simulink model "vanilla_RNN_layer"  (R2025b)
settings: Solver=ode4  StartTime=0.0  StopTime=10.0  FixedStep=1e-3  RelTol=1e-3
settings Model: Creator=llp  LastModifiedBy=llp

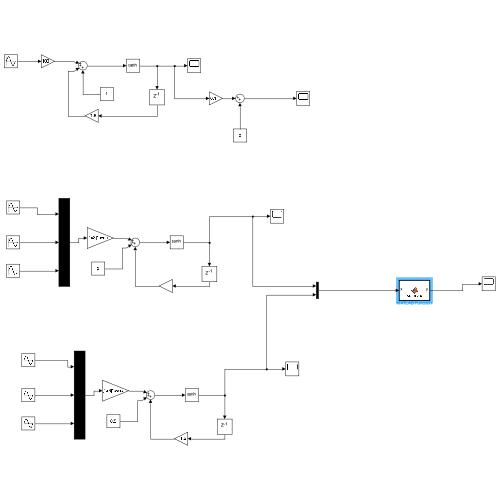
[thumbnail: Simulink's stored preview of the top-level diagram]
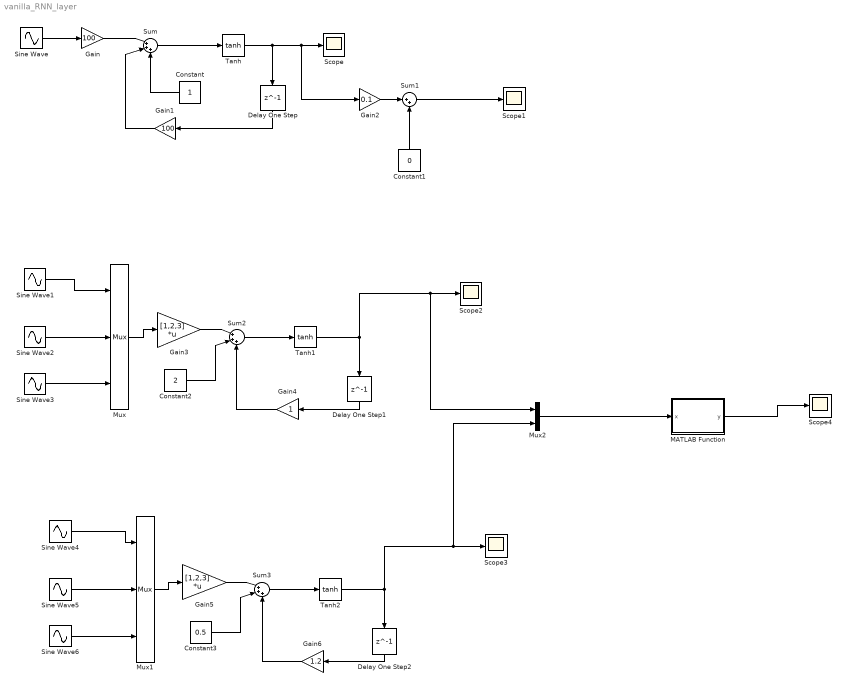
== system vanilla_RNN_layer ==
  Constant : Constant
  Constant1 : Constant  Value=0
  Constant2 : Constant  Value=2
  Constant3 : Constant  Value=0.5
  Delay One Step : Delay  DelayLength=1
  Delay One Step1 : Delay  DelayLength=1
  Delay One Step2 : Delay  DelayLength=1
  Gain : Gain  Gain=100
  Gain1 : Gain  Gain=100
  Gain2 : Gain  Gain=0.1
  Gain3 : Gain  Gain=[1,2,3]  Multiplication=Matrix(K*u) (u vector)
  Gain4 : Gain
  Gain5 : Gain  Gain=[1,2,3]  Multiplication=Matrix(K*u) (u vector)
  Gain6 : Gain  Gain=1.2
  MATLAB Function : MATLAB Function  TreatAsAtomicUnit=on
  Mux : Mux  Inputs=3
  Mux1 : Mux  Inputs=3
  Mux2 : Mux  Inputs=2
  Scope{,1..4} (5 alike) : Scope
      Scope settings: ActiveDisplayYMinimum=-1  ActiveDisplayYMaximum=1
      Scope1 settings: ActiveDisplayYMinimum=-0.125  ActiveDisplayYMaximum=0.125
      Scope2 settings: ActiveDisplayYMinimum=-1.2449101501110107  ActiveDisplayYMaximum=1.2494343446532628  DataLoggingVariableName=ScopeData2
      Scope3 settings: ActiveDisplayYMinimum=-1.2449101501110107  ActiveDisplayYMaximum=1.2494343446532628  DataLoggingVariableName=ScopeData3
      Scope4 settings: ActiveDisplayYMinimum=0.024251074532548766  ActiveDisplayYMaximum=0.9757489254674514  DataLoggingVariableName=ScopeData4
  Sine Wave : Sin  SampleTime=0
  Sine Wave1 : Sin  SampleTime=0
  Sine Wave2 : Sin  Frequency=0.6  SampleTime=0
  Sine Wave3 : Sin  Frequency=1.3  SampleTime=0
  Sine Wave4 : Sin  Frequency=0.3  SampleTime=0
  Sine Wave5 : Sin  Frequency=0.14  SampleTime=0
  Sine Wave6 : Sin  Frequency=100  SampleTime=0
  Sum : Sum  Inputs=|+++
  Sum1 : Sum  Inputs=|++
  Sum2 : Sum  Inputs=|+++
  Sum3 : Sum  Inputs=|+++
  Tanh : Trigonometry  Operator=tanh
  Tanh1 : Trigonometry  Operator=tanh
  Tanh2 : Trigonometry  Operator=tanh
  wires:
  Sine Wave/1 -> Gain/1
  Sum/1 -> Tanh/1
  Tanh/1 -> Delay One Step/1, Gain2/1, Scope/1
  Delay One Step/1 -> Gain1/1
  Constant/1 -> Sum/3
  Gain/1 -> Sum/1
  Gain1/1 -> Sum/2
  Gain2/1 -> Sum1/1
  Constant1/1 -> Sum1/2
  Sum1/1 -> Scope1/1
  Sine Wave1/1 -> Mux/1
  Sine Wave2/1 -> Mux/2
  Sine Wave3/1 -> Mux/3
  Mux/1 -> Gain3/1
  Gain3/1 -> Sum2/1
  Constant2/1 -> Sum2/2
  Sum2/1 -> Tanh1/1
  Tanh1/1 -> Delay One Step1/1, Mux2/1, Scope2/1
  Delay One Step1/1 -> Gain4/1
  Gain4/1 -> Sum2/3
  Gain5/1 -> Sum3/1
  Sine Wave4/1 -> Mux1/1
  Tanh2/1 -> Delay One Step2/1, Mux2/2, Scope3/1
  Mux1/1 -> Gain5/1
  Gain6/1 -> Sum3/3
  Sum3/1 -> Tanh2/1
  Sine Wave6/1 -> Mux1/3
  Delay One Step2/1 -> Gain6/1
  Sine Wave5/1 -> Mux1/2
  Constant3/1 -> Sum3/2
  Mux2/1 -> MATLAB Function/1(x)
  MATLAB Function/1(y) -> Scope4/1

== matlab function vanilla_RNN_layer/MATLAB Function ==
  data: x input; y output
function y = softmax_scalar(x)
%#codegen

x = x - max(x);
p = exp(x) / sum(exp(x));

y = p(1);
